simulink model "minseg_linear"  (R2024a)
settings: Solver=VariableStepAuto  StartTime=0.0  StopTime=tsim  RelTol=1e-3
values from neighbouring files (symbols this model uses):
  KLQR = lqr(A, B, Q, R)    [sim_minseg.m]
  ref = [0;0;0;0]    [sim_minseg.m]
  xs = [0;0;10/180*pi;0]    [sim_minseg.m]
undefined symbols (not defined in the file or in its folder): A, B
settings Model: Creator=Meenakshi Mahagaokar  LastModifiedBy=Meenakshi Mahagaokar
settings DataIOCC: SaveOutput=off  DSMLogging=off  SaveTime=off  ReturnWorkspaceOutputs=off

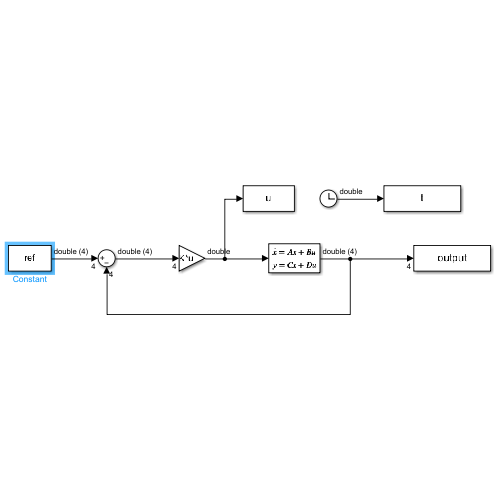
[thumbnail: Simulink's stored preview of the top-level diagram]
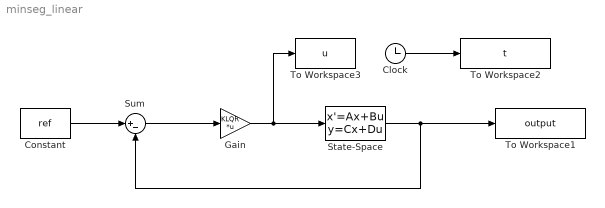
== system minseg_linear ==
  Clock : Clock
  Constant : Constant  Value=ref
  Gain : Gain  Gain=KLQR  Multiplication=Matrix(K*u)
  State-Space : StateSpace  A=A  B=B  C=[1 0 0 0; 0 1 0 0; 0 0 1 0; 0 0 0 1]  D=[0;0;0;0]  InitialCondition=xs
  Sum : Sum  Inputs=|+-
  To Workspace1 : ToWorkspace  VariableName=output  SampleTime=-1
      settings: Save2DSignal=2-D array (concatenate along first dimension)
  To Workspace2 : ToWorkspace  VariableName=t  SampleTime=-1
      settings: Save2DSignal=2-D array (concatenate along first dimension)
  To Workspace3 : ToWorkspace  VariableName=u  SampleTime=-1
      settings: Save2DSignal=2-D array (concatenate along first dimension)
  wires:
  Constant/1 -> Sum/1
  Clock/1 -> To Workspace2/1
  State-Space/1 -> Sum/2, To Workspace1/1
  Sum/1 -> Gain/1
  Gain/1 -> State-Space/1, To Workspace3/1
